simulink model "sensor_system_Interstellar"  (R2019b)
settings: Solver=VariableStepAuto  StartTime=0.0  StopTime=10.0  RelTol=1e-3
undefined symbols (not defined in the file or in its folder): gray, Rec, SDTV, strel
libraries: visionfilter x1, simulink x1, visionmorphops x1, visionanalysis x1, visionconversions x1, dspvision x1
settings Model: Creator=user  LastModifiedBy=user

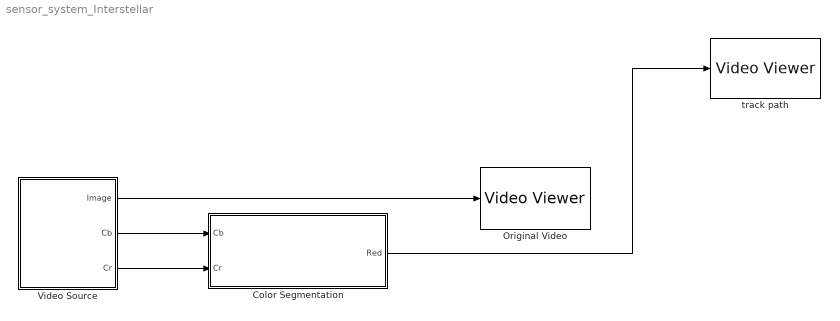
== system sensor_system_Interstellar ==
  Color Segmentation : Subsystem
  Original Video : VideoViewer  colormapValue=gray(256)  FigPos=[685 765 681 682]  trueSizedOnce=on
  "Video Source " : Subsystem
  "track path " : VideoViewer  colormapValue=gray(256)  FigPos=[1 766 683 691]  trueSizedOnce=on
  wires:
  "Video Source "/1(Image) -> Original Video/1
  Color Segmentation/1(Red) -> "track path "/1
  "Video Source "/2(Cb) -> Color Segmentation/1(Cb)
  "Video Source "/3(Cr) -> Color Segmentation/2(Cr)

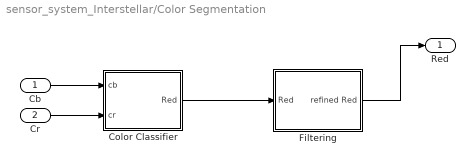
== system sensor_system_Interstellar/Color Segmentation ==
  Cb : Inport
  Cr : Inport  Port=2
  Color Classifier : Subsystem
  Filtering : Subsystem
  Red : Outport
  wires:
  Color Classifier/1("Red ") -> Filtering/1(Red)
  Cb/1 -> Color Classifier/1(cb)
  Cr/1 -> Color Classifier/2(cr)
  Filtering/1(refined Red) -> Red/1

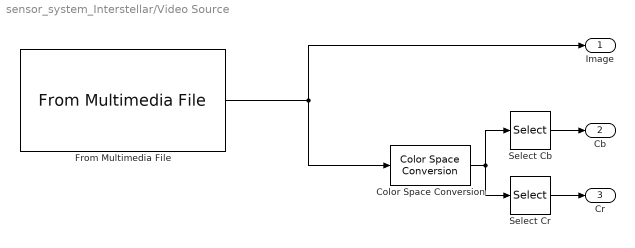
== system sensor_system_Interstellar/Video Source  ==
  Color Space Conversion : visionconversions/Color Space  Conversion  conversion=Obsolete  conversionActive=R'G'B' to Y'CbCr  wp_str=D65  rec=Rec. 601 (SDTV)  sys=1125/60/2:1  imagePorts=One multidimensional signal
  From Multimedia File : dspvision/From Multimedia File  inputFilename=C:\Users\user\Videos\2020-06-22 10-35-06.mp4  readRange=[1 Inf]  loop=on  numPlays=inf  outputStreams=Video only  videoDataType=single  audioDataType=int16  inheritSampleTime=on  userDefinedSampleTime=1/30  noAudioOutput=off  isIntensityVideo=off  fourcc=RGB  colorVideoFormat=One multidimensional signal  outputEOF=off  dataOrg=Column-major  audioFrameSize=1024  computeAudioFrameSize=off  outSamplingMode=Frame based
      settings: SourceProductName=DSP System Toolbox  SourceProductBaseCode=DS
  Select Cb : Selector  NumberOfDimensions=3  InputPortWidth=3  IndexOptions=Select all,Select all,Index vector (dialog)  Indices=[1 3],1,2  OutputSizes=1,1,1
  Select Cr : Selector  NumberOfDimensions=3  InputPortWidth=3  IndexOptions=Select all,Select all,Index vector (dialog)  Indices=[1 3],1,3  OutputSizes=1,1,1
  Image : Outport
  Cb : Outport  Port=2
  Cr : Outport  Port=3
  wires:
  Color Space Conversion/1 -> Select Cb/1, Select Cr/1
  Select Cb/1 -> Cb/1
  Select Cr/1 -> Cr/1
  From Multimedia File/1 -> Color Space Conversion/1, Image/1

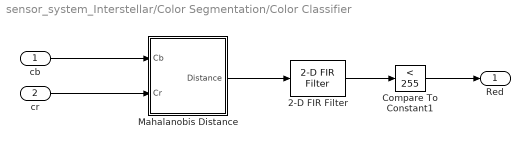
== system sensor_system_Interstellar/Color Segmentation/Color Classifier ==
  cb : Inport
  cr : Inport  Port=2
  2-D FIR Filter : visionfilter/2-D FIR Filter  separable=off  filtSrc=Specify via dialog  filterMtrx=single(1/9*ones(3))  verticalFilter=[4 0]  horizontalFilter=[4 0]  outSize=Full  padType=Constant  padSrc=Specify via dialog  padVal=0  method=Convolution  firstCoeffSignedness=Signed  firstCoeffLastDataTypeStr=Inherit: Same word length as input  outputMode=Binary point scaling  outputWordLength=32  outputFracLength=12  outputSignedness=Auto  outputLastDataTypeStr=fixdt([],32,12)  accumLastDataTypeStr=Inherit: Same as product output  prodOutputMode=Binary point scaling  prodOutputWordLength=32  prodOutputFracLength=10  prodOutputLastDataTypeStr=fixdt([],32,10)  roundingMode=Floor  overflowMode=off  firstCoeffDataTypeStr=Inherit: Same word length as input  firstCoeffMin=[]  firstCoeffMax=[]  prodOutputDataTypeStr=fixdt([],32,10)  accumDataTypeStr=Inherit: Same as product output  outputDataTypeStr=fixdt([],32,12)  outputMin=[]  outputMax=[]
      settings: SourceProductName=Computer Vision Toolbox  SourceProductBaseCode=VP
  Compare To Constant1 : simulink/Logic and Bit Operations/Compare To Constant  relop=<  const=255  OutDataTypeStr=boolean  ZeroCross=off
  "Mahalanobis Distance " : Subsystem
  "Red " : Outport
  wires:
  "Mahalanobis Distance "/1(Distance) -> 2-D FIR Filter/1
  cb/1 -> "Mahalanobis Distance "/1(Cb)
  cr/1 -> "Mahalanobis Distance "/2(Cr)
  Compare To Constant1/1 -> "Red "/1
  2-D FIR Filter/1 -> Compare To Constant1/1

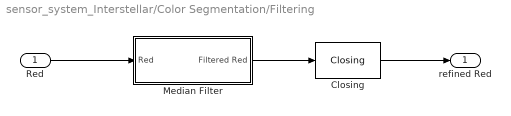
== system sensor_system_Interstellar/Color Segmentation/Filtering ==
  Red : Inport
  Closing : visionmorphops/Closing  nhoodsrc=Specify via dialog  strel=strel('disk',5)
      settings: SourceProductName=Computer Vision Toolbox  SourceProductBaseCode=VP
  Median Filter : Subsystem
  refined Red : Outport
  wires:
  Red/1 -> Median Filter/1(Red)
  Median Filter/1(Filtered Red) -> Closing/1
  Closing/1 -> refined Red/1

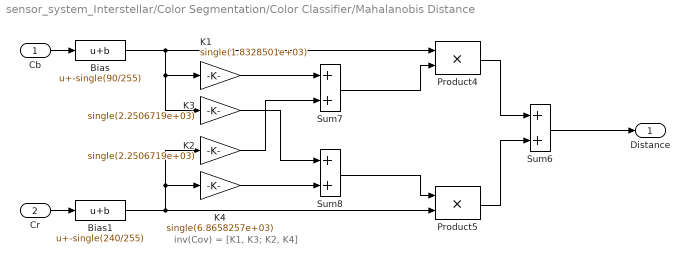
== system sensor_system_Interstellar/Color Segmentation/Color Classifier/Mahalanobis Distance  ==
  note: inv(Cov) = [K1, K3; K2, K4]
  Cb : Inport
  Cr : Inport  Port=2
  Bias : Bias  Bias=-single(90/255)
  Bias1 : Bias  Bias=-single(240/255)
  K1 : Gain  Gain=single(1.8328501e+03)  SaturateOnIntegerOverflow=on  OutDataTypeStr=Inherit: Same as input  ParamDataTypeStr=Inherit: Same as input
  K2 : Gain  Gain=single(2.2506719e+03)  SaturateOnIntegerOverflow=on  OutDataTypeStr=Inherit: Same as input  ParamDataTypeStr=Inherit: Same as input
  K3 : Gain  Gain=single(2.2506719e+03)  SaturateOnIntegerOverflow=on  OutDataTypeStr=Inherit: Same as input  ParamDataTypeStr=Inherit: Same as input
  K4 : Gain  Gain=single(6.8658257e+03)  SaturateOnIntegerOverflow=on  OutDataTypeStr=Inherit: Same as input  ParamDataTypeStr=Inherit: Same as input
  Product4 : Product  SaturateOnIntegerOverflow=on  InputSameDT=on  OutDataTypeStr=Inherit: Same as first input
  Product5 : Product  SaturateOnIntegerOverflow=on  InputSameDT=on  OutDataTypeStr=Inherit: Same as first input
  Sum6 : Sum  SaturateOnIntegerOverflow=on  InputSameDT=on  OutDataTypeStr=Inherit: Same as first input
  Sum7 : Sum  SaturateOnIntegerOverflow=on  InputSameDT=on  OutDataTypeStr=Inherit: Same as first input
  Sum8 : Sum  SaturateOnIntegerOverflow=on  InputSameDT=on  OutDataTypeStr=Inherit: Same as first input
  Distance : Outport
  wires:
  Cb/1 -> Bias/1
  Cr/1 -> Bias1/1
  K4/1 -> Sum8/2
  Product4/1 -> Sum6/1
  Product5/1 -> Sum6/2
  K1/1 -> Sum7/1
  K2/1 -> Sum7/2
  K3/1 -> Sum8/1
  Sum7/1 -> Product4/2
  Sum8/1 -> Product5/1
  Bias/1 -> Product4/1, K1/1, K3/1
  Bias1/1 -> Product5/2, K4/1, K2/1
  Sum6/1 -> Distance/1

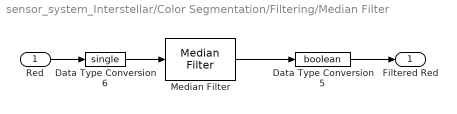
== system sensor_system_Interstellar/Color Segmentation/Filtering/Median Filter ==
  Red : Inport
  Data Type Conversion5 : DataTypeConversion  OutDataTypeStr=boolean  SaturateOnIntegerOverflow=on  RndMeth=Zero
  Data Type Conversion6 : DataTypeConversion  OutDataTypeStr=single  SaturateOnIntegerOverflow=on  RndMeth=Zero
  Median Filter : visionanalysis/Median Filter  nghbood=[3 3]  outSize=Same as input port I  padType=Constant  padSrc=Specify via dialog  padVal=0  roundingMode=Floor  overflowMode=off  prodOutputSlope=2^-30  accumSlope=2^-30  outputSlope=2^-15
      settings: SourceProductName=Computer Vision Toolbox  SourceProductBaseCode=VP
  Filtered Red : Outport
  wires:
  Red/1 -> Data Type Conversion6/1
  Data Type Conversion5/1 -> Filtered Red/1
  Median Filter/1 -> Data Type Conversion5/1
  Data Type Conversion6/1 -> Median Filter/1
